simulink model "Eq_Zeq_circuit_OLD"  (R2022b)
settings: Solver=VariableStepAuto  StartTime=0.0  StopTime=10.0  RelTol=1e-3
libraries: simrfV2elements x6, simrfV2util1 x3, simrfV2_lib x1
settings Model: Creator=umber  LastModifiedBy=umber

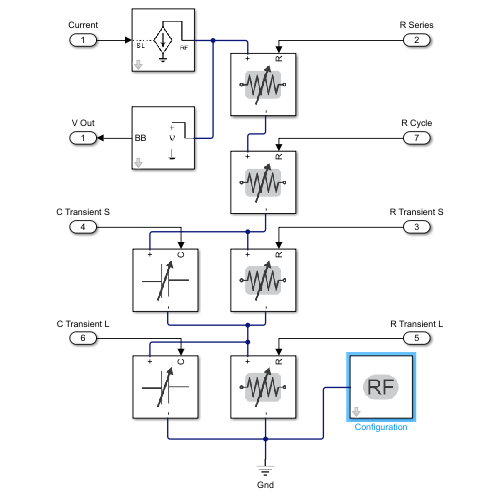
[thumbnail: Simulink's stored preview of the top-level diagram]
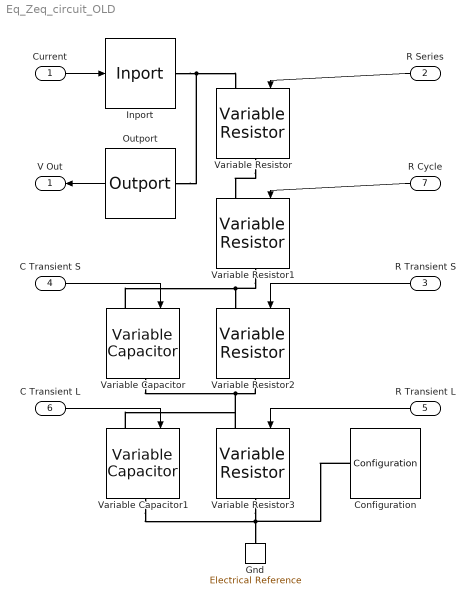
== system Eq_Zeq_circuit_OLD ==
  Current : Inport
  R Series : Inport  Port=2
  R Transient S : Inport  Port=3
  C Transient S : Inport  Port=4
  R Transient L : Inport  Port=5
  C Transient L : Inport  Port=6
  R Cycle : Inport  Port=7
  Configuration : simrfV2util1/Configuration  AutoFreq=on  Tones=[] Hz  Harmonics=[]  NormalizeCarrierPower=on  SolverType=Auto  UseCCode=on  StepSize=1e-6 s  AddNoise=on  defaultRNG=on  Seed=0  Temperature=290.0 K  SolverDelFlag=0  AbsTol=1e-6  RelTol=1e-3  MaxIter=10  ErrorEstimationType=2-norm over all variables  EnableInterpFilter=on  HiddenFIRfilterControllerParam=off  SmallSignalApprox=off  AllSimFreqs=on  SimFreqs=[] Hz  SimFreqsInternal=[]  SamplesPerFrame=1
  Gnd : simrfV2_lib/Elements/Electrical Reference
      settings: LibrarySourceBlock=simrfV2elements/Gnd  InternalSimscapePortConfiguration="{\"Bottom\":[],\"Left\":[{\"id\":\"V\",\"label\":\"\",\"type\":\"foundation.rf.circuitenvelope\"}],\"Right\":[],\"Top\":[]}"
  Inport : simrfV2util1/Inport  SimulinkInputSignalType=Ideal current  CarrierFreq=0 Hz  ZS=Inf  UseSqWave=off  NumCoeff=10  Bias=0  DutyCyc=50  InternalGrounding=on
  Outport : simrfV2util1/Outport  SensorType=Ideal voltage  OutputFormat=Complex Baseband  CarrierFreq=0 Hz  ZL=Inf  InternalGrounding=on  StepSize=1e-6 s  AutoStep=on
  Variable Capacitor : simrfV2elements/Variable Capacitor  classname=varcapacitor
  Variable Capacitor1 : simrfV2elements/Variable Capacitor  classname=varcapacitor
  Variable Resistor{,1..3} (4 alike) : simrfV2elements/Variable Resistor  classname=varresistor  hasNoise=on
  V Out : Outport
  wires:
  Current/1 -> Inport/1
  R Series/1 -> Variable Resistor/1
  Outport/1 -> V Out/1
  R Transient S/1 -> Variable Resistor2/1
  C Transient S/1 -> Variable Capacitor/1
  C Transient L/1 -> Variable Capacitor1/1
  R Transient L/1 -> Variable Resistor3/1
  R Cycle/1 -> Variable Resistor1/1
  connections:
  Variable Resistor/RConn1 -- Variable Resistor1/LConn1
  Variable Resistor1/RConn1 -- Variable Resistor2/LConn1 -- Variable Capacitor/LConn1
  Variable Capacitor/RConn1 -- Variable Capacitor1/LConn1 -- Variable Resistor3/LConn1 -- Variable Resistor2/RConn1
  Variable Capacitor1/RConn1 -- Variable Resistor3/RConn1 -- Configuration/LConn1 -- Gnd/LConn1
  Inport/RConn1 -- Outport/LConn1 -- Variable Resistor/LConn1
